simulink model "simulation"  (R2015b)
settings: Solver=VariableStepAuto  StartTime=0.0  StopTime=10.0  RelTol=1e-3
undefined symbols (not defined in the file): Ion, Lithium
libraries: powerlib x27, simulink x7, electricdrivelib x1, fuzblock x1, re_lib x1
settings Model: Creator=SPIRO-POWER  LastModifiedBy=SPIRO-POWER

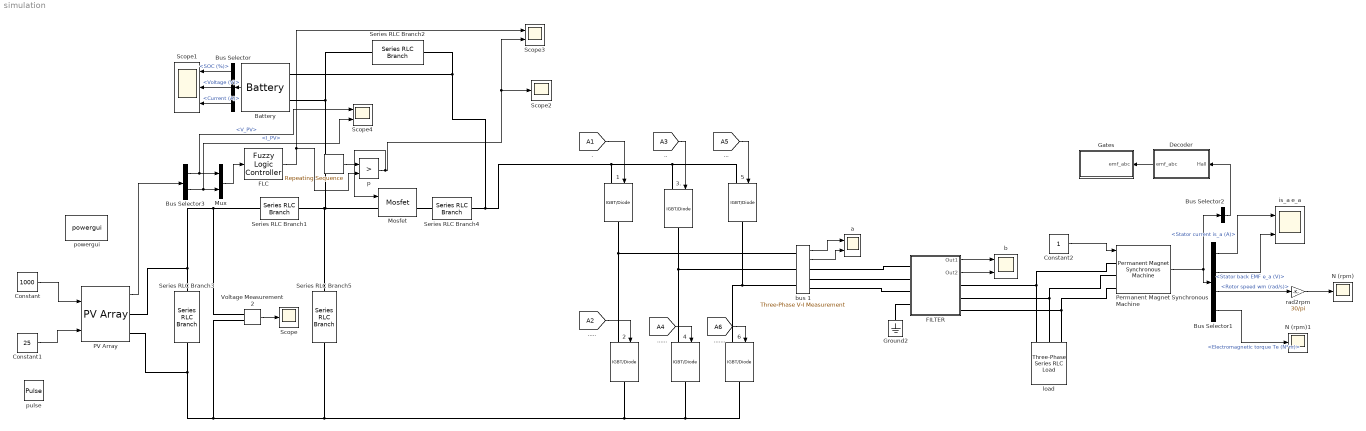
== system simulation ==
  "   " : simulink/Sources/Repeating Sequence  rep_seq_t=[0 0.0002]  rep_seq_y=[0 200]
  {1..2,4..6} (5 alike) : powerlib/Power Electronics/IGBT//Diode  Ron=1e-3  Rs=1e5  Cs=inf  Measurements=off
  3. : powerlib/Power Electronics/IGBT//Diode  Ron=1e-3  Rs=1e5  Cs=inf  Measurements=off
  Battery : electricdrivelib/Extra Sources/Battery  BatType=Lithium-Ion  ShowTempParam=off  ThermalPreset=no  NomV=12  NomQ=1.2  SOC=50  Batt_Tr=30  PresetModel=off  MaxQ=1.5  FullV=12.2  Dis_rate=2.3478  R=0.013333  Normal_OP=4.8835  expZone="[12.1     0.2653]"  current=[6.5 13 32.5]  Units=Time  Tci=20  NomT=20  T2=-30  MaxQ2=4.8  FullV2=7.1  Normal_OP2=5.72  expZone2="[6.58  1]"  Rca=0.6  ti=1000
  Bus Selector : BusSelector  OutputSignals=SOC (%),Voltage (V),Current (A)
  Bus Selector1 : BusSelector  OutputSignals=Stator current is_a (A),Stator back EMF e_a (V),Rotor speed wm (rad/s),Electromagnetic torque Te (N*m)
  Bus Selector2 : BusSelector  OutputSignals=Hall effect signal h_a,Hall effect signal h_b,Hall effect signal h_c  OutputAsBus=on
  Bus Selector3 : BusSelector  OutputSignals=V_PV,I_PV
  Constant : Constant  Value=1000
  Constant1 : Constant  Value=25
  Constant2 : Constant
  Decoder : Subsystem
  FILTER : Subsystem
  FLC : fuzblock/Fuzzy Logic  Controller  fis=anfis2
  Gates : Subsystem
  Ground2 : powerlib/Elements/Ground  LConnTagsString=a
  Mosfet : powerlib/Power Electronics/Mosfet  Ron=0.1  Lon=0  Rd=0.01  Vfd=0  IC=0  Rs=1e5  Cs=inf  Measurements=on
  Mux : Mux  Inputs=2
  N (rpm) : Scope
  N (rpm)1 : Scope
  PV Array : re_lib/Solar/PV Array  Npar=5  Nser=3  PlotType=array @ 1000 W/m2 & specified temperatures  S_vec="[ 1000  500  100 ]"  Temp_C_vec="[ 45 25  ]"  ModuleName=User-defined  PlotWhenSelected=off  Pm=80.85  Ncell=60  Voc=13  Isc=7.84  Vm=11  Im=7.35  beta_Voc_pc=-0.36099  alpha_Isc_pc=0.102  beta_Voc=-0.046929  alpha_Isc=0.0079968  IL=7.8442  I0=2.8881e-10  nI=0.35129  Rsh=89.8272  Rs=0.048032  BAL=off  Tc=1e-6  Tfilter=5e-5
  Permanent Magnet Synchronous Machine : powerlib/Machines/Permanent Magnet Synchronous Machine  NbPhases=3  FluxDistribution=Trapezoidal  RotorType=Round  MechanicalLoad=Torque Tm  PresetModel=No  ShowDetailedParameters=on  MeasurementBus=off  Resistance=1.8  Inductance=10e-3  dqInductances=[8.5e-3, 8.5e-3]  La=0.000835  MachineConstant=Flux linkage established by magnets (V.s)  Flux=0.175  VoltageCst=146.6077  TorqueCst=1.4  Flat=120  Mechanical=[ 0.8e-3, 1e-3 4]  PolePairs=4  InitialConditions=[0,0, 0,0]  InitialConditions5ph=[0 0 0 0 0 0]  TsPowergui=0  TsBlock=-1  RefAngle=90 degrees behind phase A axis (modified Park)
  Scope : Scope
  Scope1 : Scope  NumInputPorts=3
  Scope2 : Scope
  Scope3 : Scope  NumInputPorts=2
  Scope4 : Scope  NumInputPorts=2
  Series RLC Branch1 : powerlib/Elements/Series RLC Branch  LConnTagsString=__new0  RConnTagsString=__new0  BranchType=L  Resistance=1  Inductance=0.25e-3  SetiL0=off  InitialCurrent=0  Capacitance=1e-6  Setx0=off  InitialVoltage=0  Measurements=None
  Series RLC Branch2 : powerlib/Elements/Series RLC Branch  LConnTagsString=__new0  RConnTagsString=__new0  BranchType=C  Resistance=1  Inductance=1e-3  SetiL0=off  InitialCurrent=0  Capacitance=100e-6  Setx0=off  InitialVoltage=0  Measurements=Branch voltage
  Series RLC Branch3 : powerlib/Elements/Series RLC Branch  LConnTagsString=__new0  RConnTagsString=__new0  BranchType=C  Resistance=1  Inductance=1e-3  SetiL0=off  InitialCurrent=0  Capacitance=100e-6  Setx0=off  InitialVoltage=0  Measurements=Branch voltage
  Series RLC Branch4 : powerlib/Elements/Series RLC Branch  LConnTagsString=__new0  RConnTagsString=__new0  BranchType=L  Resistance=1  Inductance=10e-3  SetiL0=off  InitialCurrent=0  Capacitance=1e-6  Setx0=off  InitialVoltage=0  Measurements=None
  Series RLC Branch5 : powerlib/Elements/Series RLC Branch  LConnTagsString=__new0  RConnTagsString=__new0  BranchType=C  Resistance=1  Inductance=1e-3  SetiL0=off  InitialCurrent=0  Capacitance=100e-6  Setx0=off  InitialVoltage=0  Measurements=Branch voltage
  Voltage Measurement2 : powerlib/Measurements/Voltage Measurement  PhasorSimulation=off  OutputType=Complex  PSBequivalent=0
  a : Scope  NumInputPorts=2
  b : Scope  NumInputPorts=2
  bus 1 : powerlib/Measurements/Three-Phase V-I Measurement  VoltageMeasurement=phase-to-ground  SetLabelV=off  LabelV=Vabc  Vpu=off  VpuLL=off  CurrentMeasurement=yes  SetLabelI=off  LabelI=Iabc  Ipu=off  Pbase=100e6  Vbase=500e3  OutputType=Complex  PhasorSimulation=off  PSBequivalent=0
  is_a e_a : Scope  NumInputPorts=2
  load : powerlib/Elements/Three-Phase Series RLC Load  LConnTagsString=A|B|C  Configuration=Y (grounded)  NominalVoltage=1000  Vabc=[1e3 1e3 1e3]  Vabcp=[1e3 1e3 1e3]  NominalFrequency=60  UnbalancedPower=off  ActivePower=10e3  InductivePower=0  CapacitivePower=0  Pabc=[10e3 9e3 11e3]  QLabc=[100 90 110]  QCabc=[100 90 110]  Pabcp=[10e3 9e3 11e3]  QLabcp=[100 90 110]  QCabcp=[100 90 110]  Measurements=None  LoadType=constant Z
  p : RelationalOperator  Operator=>  OutDataTypeStr=boolean
  powergui : powerlib/powergui  Priority=1  SimulationMode=Discrete  SolverType=Tustin  SampleTime=5e-6  frequency=60  SPID=off  DisableSnubberDevices=off  DisableRonSwitches=off  DisableVfSwitches=off  SwTol=0  DisplayEquations=off  Interpol=off  ExternalGateDelay=off  methode=off  Ts=10  FunctionMessages=off  echomessages=off  HookPort=off  EnableUseOfTLC=off  x0status=blocks  frequencyindice=0  Pbase=100e6  ErrMax=1e-4  Iterations=50  UnitsV=kV  UnitsW=MW  buscounter=0  RestoreLinks=warning  ResistiveCurrentMeasurement=off  Frange=[0:2:500]  Ylog=off  Xlog=on  ShowGrid=off  save=off  variable=ZData  structure=0  ZoomFFT=off  StartTime=0.0  cycles=1  DisplayStyle=1  fundamental=60  FreqAxis=off  MaxFrequency=1000  frequencyindicesteady=1  RmsSteady=1  display=off
  "pulse " : DiscretePulseGenerator  PulseType=Time based  Period=0.0002  PulseWidth=50
  rad2rpm : Gain  Gain=30/pi
  wires:
  Battery/1 -> Bus Selector/1
  Bus Selector/2 -> Scope1/2  "<Voltage (V)>"
  Bus Selector/3 -> Scope1/3  "<Current (A)>"
  Bus Selector/1 -> Scope1/1  "<SOC (%)>"
  [A1] -> 1/1
  [A3] -> 3./1
  [A5] -> 5/1
  [A2] -> 2/1
  [A4] -> 4/1
  [A6] -> 6/1
  Constant2/1 -> Permanent Magnet Synchronous Machine/1
  Decoder/1(emf_abc) -> Gates/1("emf_abc ")
  rad2rpm/1 -> N (rpm)/1
  Bus Selector1/1 -> is_a e_a/1  "<Stator current is_a (A)>"
  Permanent Magnet Synchronous Machine/1 -> Bus Selector1/1, Bus Selector2/1
  Bus Selector2/1 -> Decoder/1("Hall ")
  Bus Selector1/2 -> is_a e_a/2  "<Stator back EMF e_a (V)>"
  Bus Selector1/3 -> rad2rpm/1  "<Rotor speed wm (rad/s)>"
  Bus Selector1/4 -> N (rpm)1/1  "<Electromagnetic torque Te (N*m)>"
  bus 1/1 -> a/1
  bus 1/2 -> a/2
  Constant/1 -> PV Array/1
  Constant1/1 -> PV Array/2
  FILTER/1(Out1) -> b/1
  FILTER/2(Out2) -> b/2
  Voltage Measurement2/1 -> Scope/1
  FLC/1 -> p/2, Scope3/1
  Mux/1 -> FLC/1
  PV Array/1 -> Bus Selector3/1
  Bus Selector3/1 -> Scope4/1, Mux/1  "<V_PV>"
  Bus Selector3/2 -> Scope4/2, Mux/2  "<I_PV>"
  "   "/1 -> p/1
  p/1 -> Mosfet/1, Scope2/1, Scope3/2
  connections:
  PV Array/RConn2 -- Voltage Measurement2/LConn2 -- 2/RConn1 -- 6/RConn1 -- 4/RConn1 -- Series RLC Branch5/RConn1 -- Series RLC Branch3/RConn1
  Battery/LConn1 -- Series RLC Branch2/LConn1 -- 5/LConn1 -- 3./LConn1 -- 1/LConn1 -- Series RLC Branch4/RConn1
  bus 1/LConn1 -- 2/LConn1 -- 1/RConn1
  bus 1/LConn2 -- 4/LConn1 -- 3./RConn1
  bus 1/LConn3 -- 6/LConn1 -- 5/RConn1
  load/LConn2 -- Permanent Magnet Synchronous Machine/LConn2 -- FILTER/RConn2
  Permanent Magnet Synchronous Machine/LConn3 -- FILTER/RConn3 -- load/LConn3
  Series RLC Branch2/RConn1 -- Battery/LConn2 -- Mosfet/LConn1 -- Series RLC Branch5/LConn1 -- Series RLC Branch1/RConn1
  PV Array/RConn1 -- Voltage Measurement2/LConn1 -- Series RLC Branch1/LConn1 -- Series RLC Branch3/LConn1
  Mosfet/RConn1 -- Series RLC Branch4/LConn1
  Permanent Magnet Synchronous Machine/LConn1 -- FILTER/RConn1 -- load/LConn1
  FILTER/LConn1 -- bus 1/RConn1
  FILTER/LConn2 -- bus 1/RConn2
  FILTER/LConn3 -- bus 1/RConn3
  Ground2/LConn1 -- FILTER/LConn4

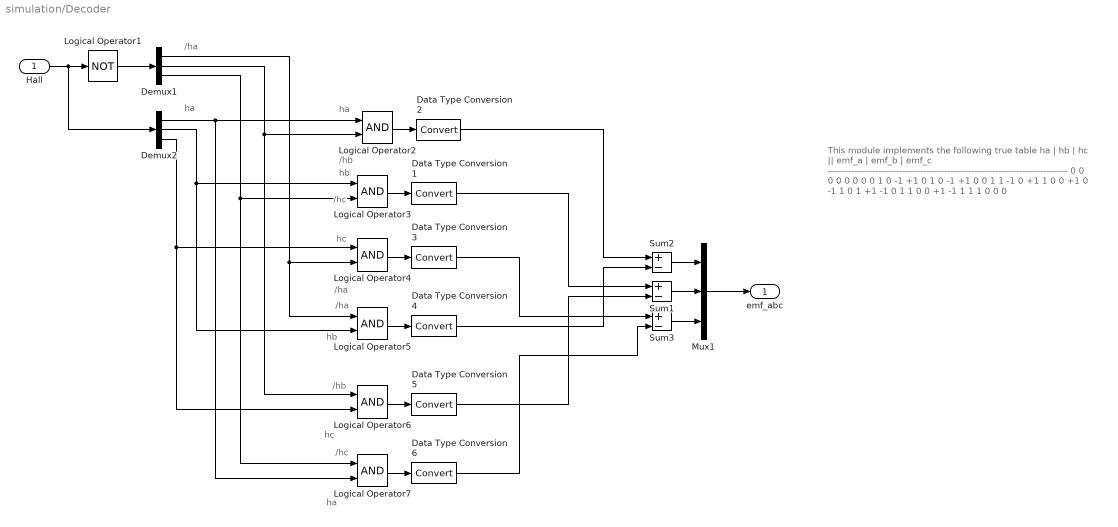
== system simulation/Decoder ==
  note: /ha
  note: ha
  note: ha
  note: /hb
  note: hb
  note: /hc
  note: hc
  note: /ha
  note: /ha
  note: hb
  note: /hb
  note: hc
  note: /hc
  note: ha
  note: This module implements the following true table
      |
      |    ha   |   hb   |   hc   ||   emf_a   |   emf_b   |   emf_c
      |     --------------------------------------------------------------------------------
      | 0          0         0          0               0               0
      | 0          0         1          0               -1              +1
      | 0          1         0          -1              +1                0
      | 0          1         1          -1               0               +1
      | 1          0         0         +1               0               -1
      | 1          0         1         +1              -1                0
      | 1          1         0          0              +1               -1
      | 1          1         1          0               0                0
  "Hall " : Inport
  Data Type Conversion{1..6} (6 alike) : DataTypeConversion
  Demux1 : Demux  Outputs=3
  Demux2 : Demux  Outputs=3
  Logical Operator1 : Logic  Operator=NOT  AllPortsSameDT=off  OutDataTypeStr=boolean
  Logical Operator{2..7} (6 alike) : Logic  AllPortsSameDT=off  OutDataTypeStr=boolean
  Mux1 : Mux  Inputs=3
  Sum1 : Sum  Inputs=+-  OutDataTypeStr=double
  Sum2 : Sum  Inputs=+-  OutDataTypeStr=double
  Sum3 : Sum  Inputs=+-  OutDataTypeStr=double
  emf_abc : Outport
  wires:
  "Hall "/1 -> Logical Operator1/1, Demux2/1
  Logical Operator1/1 -> Demux1/1
  Demux2/3 -> Logical Operator4/1, Logical Operator6/2
  Demux2/2 -> Logical Operator3/1, Logical Operator5/2
  Demux2/1 -> Logical Operator2/1, Logical Operator7/2
  Demux1/3 -> Logical Operator3/2, Logical Operator7/1
  Demux1/2 -> Logical Operator2/2, Logical Operator6/1
  Demux1/1 -> Logical Operator4/2, Logical Operator5/1
  Logical Operator2/1 -> Data Type Conversion2/1
  Sum2/1 -> Mux1/1
  Sum1/1 -> Mux1/2
  Sum3/1 -> Mux1/3
  Mux1/1 -> emf_abc/1
  Logical Operator3/1 -> Data Type Conversion1/1
  Logical Operator4/1 -> Data Type Conversion3/1
  Logical Operator5/1 -> Data Type Conversion4/1
  Logical Operator6/1 -> Data Type Conversion5/1
  Logical Operator7/1 -> Data Type Conversion6/1
  Data Type Conversion2/1 -> Sum2/1
  Data Type Conversion4/1 -> Sum2/2
  Data Type Conversion1/1 -> Sum1/1
  Data Type Conversion5/1 -> Sum1/2
  Data Type Conversion3/1 -> Sum3/1
  Data Type Conversion6/1 -> Sum3/2

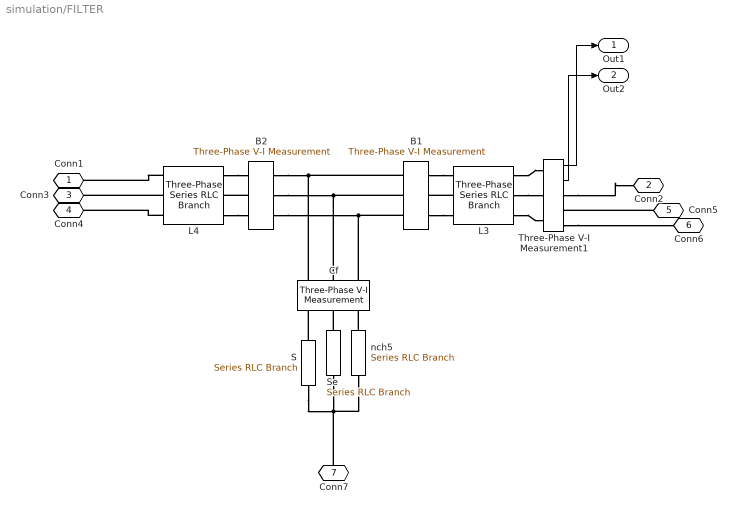
== system simulation/FILTER ==
  B1 : powerlib/Measurements/Three-Phase V-I Measurement  VoltageMeasurement=phase-to-ground  SetLabelV=on  LabelV=UL  Vpu=off  VpuLL=off  CurrentMeasurement=yes  SetLabelI=on  LabelI=IL  Ipu=off  Pbase=3.6e6  Vbase=0.69e3  OutputType=Magnitude  PhasorSimulation=off  PSBequivalent=0
  B2 : powerlib/Measurements/Three-Phase V-I Measurement  VoltageMeasurement=phase-to-ground  SetLabelV=on  LabelV=ULC  Vpu=off  VpuLL=off  CurrentMeasurement=yes  SetLabelI=on  LabelI=ILC  Ipu=off  Pbase=3.6e6  Vbase=0.69e3  OutputType=Magnitude  PhasorSimulation=off  PSBequivalent=0
  Cf : powerlib/Measurements/Three-Phase V-I Measurement  VoltageMeasurement=phase-to-ground  SetLabelV=on  LabelV=Uf  Vpu=off  VpuLL=off  CurrentMeasurement=yes  SetLabelI=on  LabelI=If  Ipu=off  Pbase=100e6  Vbase=500e3  OutputType=Magnitude  PhasorSimulation=off  PSBequivalent=0
  L3 : powerlib/Elements/Three-Phase Series RLC Branch  LConnTagsString=A|B|C  RConnTagsString=A|B|C  BranchType=RL  Resistance=0.1667  Inductance=1.5321e-3  Capacitance=inf  Measurements=None
  L4 : powerlib/Elements/Three-Phase Series RLC Branch  LConnTagsString=A|B|C  RConnTagsString=A|B|C  BranchType=RL  Resistance=0.0096  Inductance=1.5321e-3  Capacitance=inf  Measurements=None
  S : powerlib/Elements/Series RLC Branch  LConnTagsString=__new0  RConnTagsString=__new0  BranchType=RC  Resistance=0.3462  Inductance=1e-3  SetiL0=off  InitialCurrent=0  Capacitance=3.1022e-4  Setx0=off  InitialVoltage=0  Measurements=None
  Se : powerlib/Elements/Series RLC Branch  LConnTagsString=__new0  RConnTagsString=__new0  BranchType=RC  Resistance=0.3462  Inductance=1e-3  SetiL0=off  InitialCurrent=0  Capacitance=3.1022e-4  Setx0=off  InitialVoltage=0  Measurements=None
  Three-Phase V-I Measurement1 : powerlib/Measurements/Three-Phase V-I Measurement  VoltageMeasurement=phase-to-phase  SetLabelV=off  LabelV=Vabc  Vpu=off  VpuLL=off  CurrentMeasurement=yes  SetLabelI=off  LabelI=Iabc  Ipu=off  Pbase=100e6  Vbase=500e3  OutputType=Complex  PhasorSimulation=off  PSBequivalent=0
  nch5 : powerlib/Elements/Series RLC Branch  LConnTagsString=__new0  RConnTagsString=__new0  BranchType=RC  Resistance=0.3462  Inductance=1e-3  SetiL0=off  InitialCurrent=0  Capacitance=3.1022e-4  Setx0=off  InitialVoltage=0  Measurements=None
  Conn1 : PMIOPort  Port=1  Side=Left
  Conn2 : PMIOPort  Port=2  Side=Right
  Conn3 : PMIOPort  Port=3  Side=Left
  Conn4 : PMIOPort  Port=4  Side=Left
  Conn5 : PMIOPort  Port=5  Side=Right
  Conn6 : PMIOPort  Port=6  Side=Right
  Conn7 : PMIOPort  Port=7  Side=Left
  Out1 : Outport
  Out2 : Outport  Port=2
  wires:
  Three-Phase V-I Measurement1/1 -> Out1/1
  Three-Phase V-I Measurement1/2 -> Out2/1
  connections:
  Three-Phase V-I Measurement1/RConn3 -- Conn6/RConn1
  Conn5/RConn1 -- Three-Phase V-I Measurement1/RConn2
  Three-Phase V-I Measurement1/RConn1 -- Conn2/RConn1
  Se/RConn1 -- Conn7/RConn1 -- S/RConn1 -- nch5/RConn1
  Cf/LConn1 -- B1/LConn1 -- B2/RConn1
  Cf/LConn2 -- B1/LConn2 -- B2/RConn2
  Cf/LConn3 -- B1/LConn3 -- B2/RConn3
  L4/LConn3 -- Conn4/RConn1
  B1/RConn3 -- L3/LConn3
  L3/RConn2 -- Three-Phase V-I Measurement1/LConn2
  L4/RConn1 -- B2/LConn1
  L3/RConn3 -- Three-Phase V-I Measurement1/LConn3
  L4/RConn3 -- B2/LConn3
  B1/RConn1 -- L3/LConn1
  nch5/LConn1 -- Cf/RConn3
  L3/LConn2 -- B1/RConn2
  Se/LConn1 -- Cf/RConn2
  L3/RConn1 -- Three-Phase V-I Measurement1/LConn1
  S/LConn1 -- Cf/RConn1
  L4/LConn1 -- Conn1/RConn1
  L4/LConn2 -- Conn3/RConn1
  B2/LConn2 -- L4/RConn2

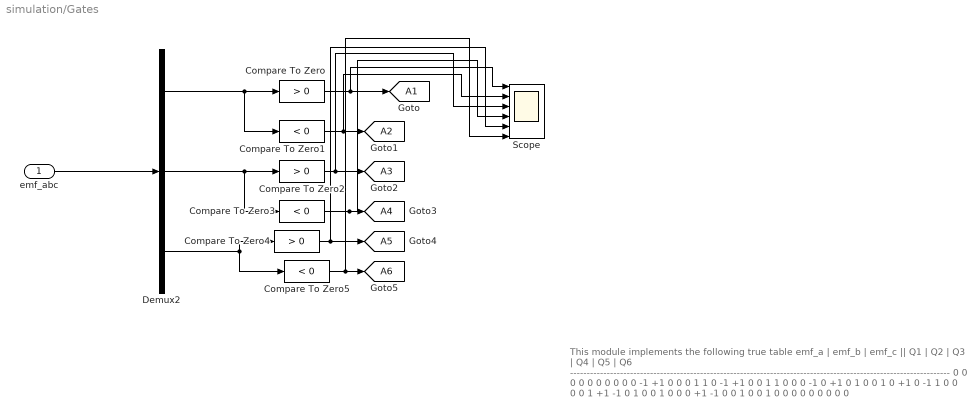
== system simulation/Gates ==
  note: This module implements the following true table
      |
      |    emf_a   |   emf_b   |   emf_c   ||   Q1   |   Q2   |   Q3   |   Q4   |   Q5   |   Q6
      |     ------------------------------------------------------------------------------------------------------------------
      |       0              0                0            0          0          0           0        0        0
      |       0               -1              +1          0          0          0           1        1        0
      |     -1              +1                0          0          1          1           0        0        0
      |     -1               0               +1          0          1         0           0        1        0
      |    +1               0                -1          1          0          0           0        0        1
      |    +1              -1                0           1          0          0           1        0        0
      |      0              +1               -1           0          0          1           0        0        1
      |     0              0                0             0          0          0           0        0        0
  "emf_abc " : Inport
  Compare To Zero : simulink/Logic and Bit Operations/Compare To Zero  relop=>  OutDataTypeStr=boolean  ZeroCross=off
  Compare To Zero1 : simulink/Logic and Bit Operations/Compare To Zero  relop=<  OutDataTypeStr=boolean  ZeroCross=off
  Compare To Zero2 : simulink/Logic and Bit Operations/Compare To Zero  relop=>  OutDataTypeStr=boolean  ZeroCross=off
  Compare To Zero3 : simulink/Logic and Bit Operations/Compare To Zero  relop=<  OutDataTypeStr=boolean  ZeroCross=off
  Compare To Zero4 : simulink/Logic and Bit Operations/Compare To Zero  relop=>  OutDataTypeStr=boolean  ZeroCross=off
  Compare To Zero5 : simulink/Logic and Bit Operations/Compare To Zero  relop=<  OutDataTypeStr=boolean  ZeroCross=off
  Demux2 : Demux  Outputs=3
  Scope : Scope  NumInputPorts=6
  tag scope: A1=global, A2=global, A3=global, A4=global, A5=global, A6=global
  wires:
  "emf_abc "/1 -> Demux2/1
  Demux2/1 -> Compare To Zero/1, Compare To Zero1/1
  Demux2/2 -> Compare To Zero2/1, Compare To Zero3/1
  Demux2/3 -> Compare To Zero4/1, Compare To Zero5/1
  Compare To Zero/1 -> Scope/1, [A1]
  Compare To Zero1/1 -> Scope/2, [A2]
  Compare To Zero2/1 -> Scope/3, [A3]
  Compare To Zero3/1 -> Scope/4, [A4]
  Compare To Zero4/1 -> [A5], Scope/5
  Compare To Zero5/1 -> Scope/6, [A6]
